simulink model "mpu6050_kalman_verification"  (R2014a)
settings: Solver=ode45  StartTime=0.0  StopTime=20  RelTol=1e-3
libraries: commnoisgen2 x1
settings Model: Creator=Administrator  LastModifiedBy=Administrator

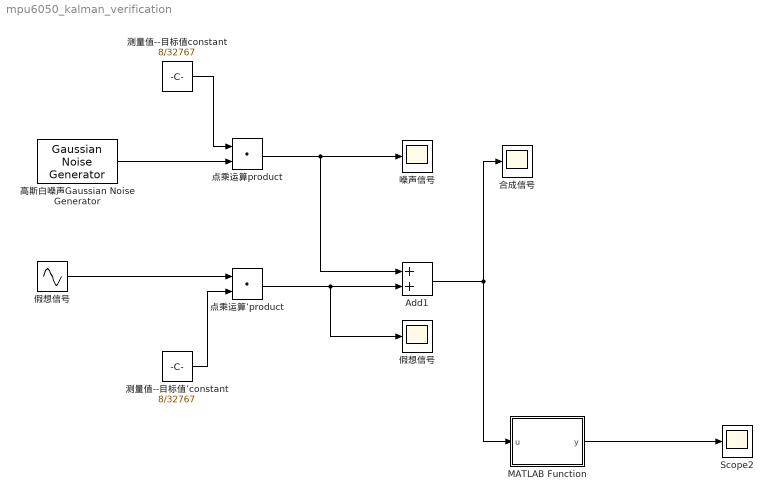
== system mpu6050_kalman_verification ==
  Add1 : Sum  SampleTime=0.001
  MATLAB Function : MATLAB Function  TreatAsAtomicUnit=on
  Scope2 : Scope
      settings: SaveName=ScopeData2
  假想信号 : Sin  Amplitude=20  Frequency=100  SampleTime=0.001
  "假想信号 " : Scope
      settings: SaveName=ScopeData3
  合成信号 : Scope
  噪声信号 : Scope
  测量值--目标值constant : Constant  Value=8/32767  SampleTime=0.001
  测量值--目标值’constant : Constant  Value=8/32767  SampleTime=0.001
  点乘运算product : DotProduct  InputSameDT=on  OutDataTypeStr=Inherit: Inherit via internal rule
  点乘运算‘product : DotProduct  InputSameDT=on  OutDataTypeStr=Inherit: Inherit via internal rule
  高斯白噪声Gaussian Noise Generator : commnoisgen2/Gaussian Noise Generator  m=0  d=11.7806  s=0  Ts=0.001  frameBased=off  sampPerFrame=1  orient=off  outDataType=double
  wires:
  Add1/1 -> 合成信号/1, MATLAB Function/1(u)
  MATLAB Function/1(y) -> Scope2/1
  高斯白噪声Gaussian Noise Generator/1 -> 点乘运算product/2
  点乘运算product/1 -> Add1/1, 噪声信号/1
  点乘运算‘product/1 -> "假想信号 "/1, Add1/2
  测量值--目标值constant/1 -> 点乘运算product/1
  测量值--目标值’constant/1 -> 点乘运算‘product/2
  假想信号/1 -> 点乘运算‘product/1

== matlab function mpu6050_kalman_verification/MATLAB Function ==
  data: u input; y output
function y = kalman(u)
%#codegen



y = u;
